simulink model "sldemo_absbrake_ATESST"  (Simulink 7.4)
settings: Solver=ode45  StartTime=0.0  StopTime=15  RelTol=1e-3
settings Model: Creator=carlj  LastModifiedBy=alesch
settings OptimizationCC: InlineParams=on
settings DebuggingCC: StrictBusMsg=ErrorLevel1

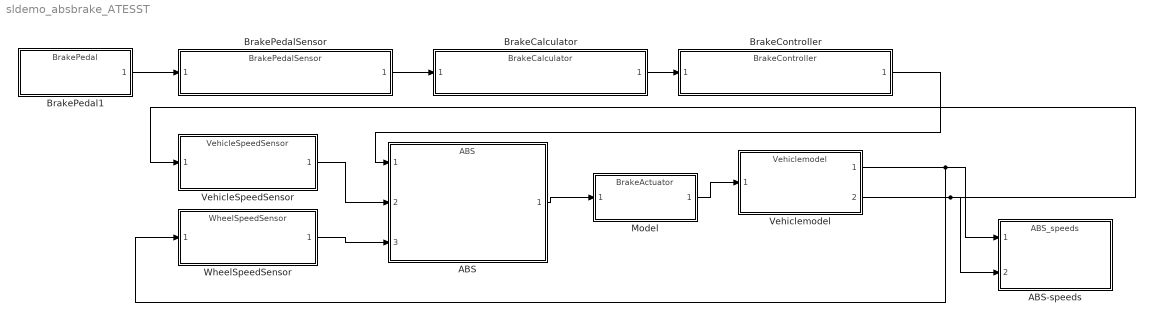
== system sldemo_absbrake_ATESST ==
  ABS : ModelReference  ModelNameDialog=ABS  SimulationMode=Accelerator  ModelReferenceVersion=1.16  CopyOfModelName=ABS
  ABS-speeds : ModelReference  ModelNameDialog=ABS_speeds  SimulationMode=Accelerator  ModelReferenceVersion=1.12  CopyOfModelName=ABS_speeds
  BrakeCalculator : ModelReference  ModelNameDialog=BrakeCalculator  SimulationMode=Accelerator  ModelReferenceVersion=1.15  CopyOfModelName=BrakeCalculator
  BrakeController : ModelReference  ModelNameDialog=BrakeController  SimulationMode=Accelerator  ModelReferenceVersion=1.15  CopyOfModelName=BrakeController
  BrakePedal1 : ModelReference  ModelNameDialog=BrakePedal  SimulationMode=Accelerator  ModelReferenceVersion=1.14  CopyOfModelName=BrakePedal
  BrakePedalSensor : ModelReference  ModelNameDialog=BrakePedalSensor  SimulationMode=Accelerator  ModelReferenceVersion=1.16  CopyOfModelName=BrakePedalSensor
  Model : ModelReference  ModelNameDialog=BrakeActuator  SimulationMode=Accelerator  ModelReferenceVersion=1.1  CopyOfModelName=BrakeActuator
  VehicleSpeedSensor : ModelReference  ModelNameDialog=VehicleSpeedSensor  SimulationMode=Accelerator  ModelReferenceVersion=1.17  CopyOfModelName=VehicleSpeedSensor
  Vehiclemodel : ModelReference  ModelNameDialog=Vehiclemodel  SimulationMode=Accelerator  ModelReferenceVersion=1.17  CopyOfModelName=Vehiclemodel
  "WheelSpeedSensor " : ModelReference  ModelNameDialog=WheelSpeedSensor  SimulationMode=Accelerator  ModelReferenceVersion=1.17  CopyOfModelName=WheelSpeedSensor
  wires:
  Vehiclemodel/2 -> VehicleSpeedSensor/1, ABS-speeds/2
  BrakePedalSensor/1 -> BrakeCalculator/1
  BrakeCalculator/1 -> BrakeController/1
  BrakePedal1/1 -> BrakePedalSensor/1
  Vehiclemodel/1 -> ABS-speeds/1, "WheelSpeedSensor "/1
  ABS/1 -> Model/1
  Model/1 -> Vehiclemodel/1
  "WheelSpeedSensor "/1 -> ABS/3
  VehicleSpeedSensor/1 -> ABS/2
  BrakeController/1 -> ABS/1
